simulink model "nichtl_1"  (Simulink 4.00)
settings: Solver=ode113  SolverMode=SingleTasking  StartTime=0.0  StopTime=0.05  FixedStep=1e-6  MaxStep=5e-5  RelTol=1e-3  AbsTol=1e-6
values from neighbouring files (symbols this model uses):
  C = 500e-6    (= 0.0005)    [inv_switch_1.m]    (also in mehrw_1.m = eye(10,10); mehrw_2.m = eye(10,10); mehrw_3.m = eye(10,10); mehrw_4.m = eye(10,10))
  fs = 1/d_t    (= 100)    [fmasse_var_1.m]    (also in fmasse_var_2.m; pnichtl1.m = 5000; pnichtl2.m = 5000)
  I0 = 20e-9    (= 2e-08)    [pnichtl1.m]    (also in pnichtl2.m)
  R = 100e3    (= 100000)    [pnichtl1.m]    (also in pnichtl2.m)
  Rg = 10e3    (= 10000)    [pnichtl1.m]    (also in pnichtl2.m)
  VT = 25e-3    (= 0.025)    [pnichtl1.m]    (also in pnichtl2.m)
settings Model: LastModifiedBy=Administrator  MaxDataPoints=2500  ExtModeTrigMode=oneshot  ExtModeArmWhenConnect=off  BlockReductionOpt=off

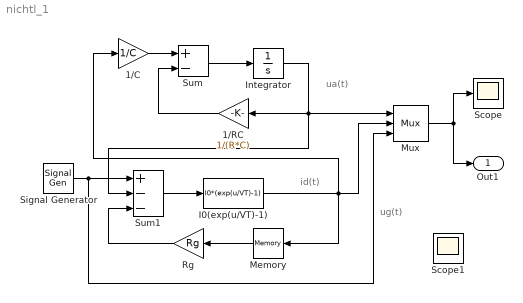
== system nichtl_1 ==
  note: ua(t)
  note: id(t)
  note: ug(t)
  1/C : Gain  Gain=1/C  Multiplication=Element-wise(K.*u)  SaturateOnIntegerOverflow=on
  1/RC : Gain  Orientation=left  Gain=1/(R*C)  Multiplication=Element-wise(K.*u)  SaturateOnIntegerOverflow=on
  I0(exp(u/VT)-1) : Fcn  Expr=I0*(exp(u/VT)-1)
  Integrator : Integrator  ExternalReset=none  InitialConditionSource=internal  InitialCondition=0  LimitOutput=off  UpperSaturationLimit=inf  LowerSaturationLimit=-inf  ShowSaturationPort=off  ShowStatePort=off  AbsoluteTolerance=auto
  Memory : Memory  Orientation=left  X0=0  InheritSampleTime=off
  Mux : Mux  Inputs=3
      settings: DisplayOption=none
  Rg : Gain  Orientation=left  Gain=Rg  Multiplication=Element-wise(K.*u)  SaturateOnIntegerOverflow=on
  Scope : Scope
      settings: TickLabels=on  TimeRange=0.001  YMin=-1  YMax=1  SaveToWorkspace=off  SaveName=ScopeData  DataFormat=Array  LimitDataPoints=on  MaxDataPoints=5000
  Scope1 : Scope
      settings: Floating=on  TickLabels=on  TimeRange=0.001  YMin=-5e-005  YMax=0.00035  SaveToWorkspace=off  SaveName=ScopeData  DataFormat=Array  LimitDataPoints=on  MaxDataPoints=5000
  Signal Generator : SignalGenerator  WaveForm=sine  Amplitude=1  Frequency=fs  Units=Hertz
  Sum : Sum  Inputs=+-  SaturateOnIntegerOverflow=on
  Sum1 : Sum  Inputs=+--  SaturateOnIntegerOverflow=on
  Out1 : Outport  Port=1
  wires:
  1/C/1 -> Sum/1
  Sum/1 -> Integrator/1
  1/RC/1 -> Sum/2
  Sum1/1 -> I0(exp(u/VT)-1)/1
  Rg/1 -> Sum1/3
  Integrator/1 -> 1/RC/1, Sum1/2, Mux/1
  Memory/1 -> Rg/1
  I0(exp(u/VT)-1)/1 -> 1/C/1, Memory/1, Mux/2
  Signal Generator/1 -> Sum1/1, Mux/3
  Mux/1 -> Scope/1, Out1/1
